simulink model "Linear_Model_Ters_Sarkac"  (R2022a)
settings: Solver=ode4  StartTime=0.0  StopTime=20  FixedStep=1/1000  RelTol=1e-3
InitFcn:
  | Sarkac_Parametrelerini_Yukle
values from neighbouring files (symbols this model uses):
  A = [0      1              0           0 ... (first row only)    [Sarkac_Parametrelerini_Yukle.m]
  B = [     0 ... (first row only)    [Sarkac_Parametrelerini_Yukle.m]
  Baslangic_Degerleri_Lin = [0,0,deg2rad(15),0]    [Sarkac_Parametrelerini_Yukle.m]
  C = eye(4)    [Sarkac_Parametrelerini_Yukle.m]
  D = zeros(4,1)    [Sarkac_Parametrelerini_Yukle.m]
  LQR_Katsayi_Matrisi = K    [Sarkac_Parametrelerini_Yukle.m]
libraries: simulink_extras x2, vrlib x1
settings Model: Creator=Fatabi  LastModifiedBy=Fatabi
settings SolverCC: AlgebraicLoopSolver=TrustRegion
settings DebuggingCC: UnconnectedInputMsg=warning  UnconnectedOutputMsg=warning  UnconnectedLineMsg=warning  SFMachineParentedDataDiag=warning

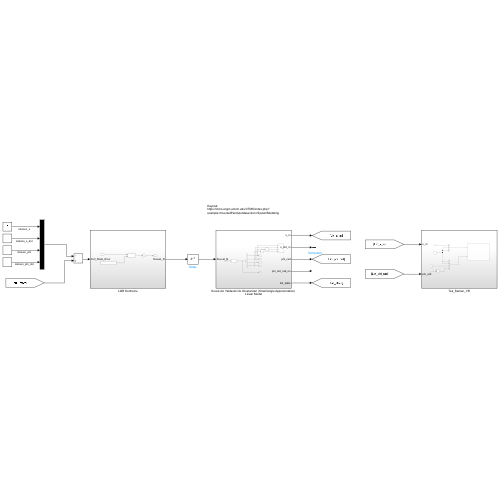
[thumbnail: Simulink's stored preview of the top-level diagram]
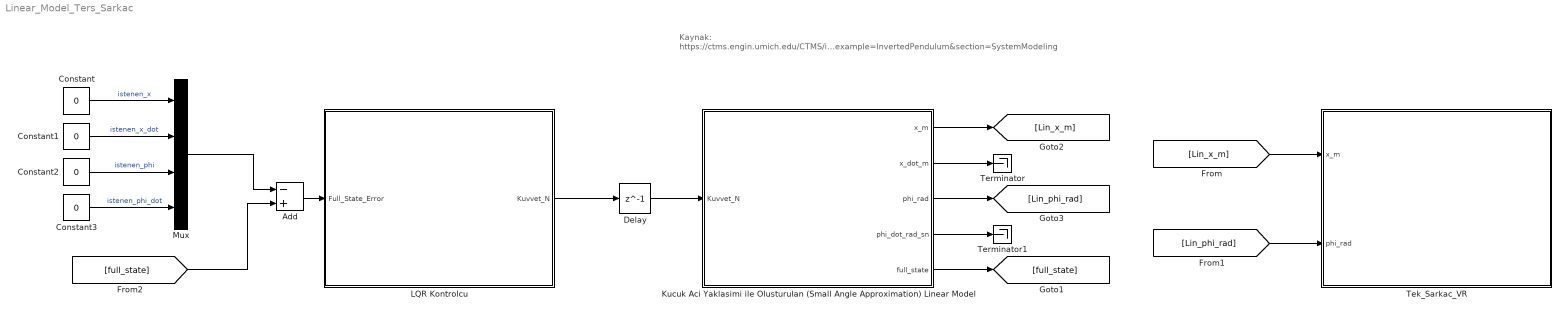
== system Linear_Model_Ters_Sarkac ==
  note: Kaynak:
      | https://ctms.engin.umich.edu/CTMS/index.php?example=InvertedPendulum&section=SystemModeling
  Add : Sum  Inputs=-+
  Constant{,1..3} (4 alike) : Constant  Value=0
  Delay : Delay  DelayLength=1
  Kucuk Aci Yaklasimi ile Olusturulan (Small Angle Approximation) Linear Model : Subsystem
  LQR Kontrolcu : Subsystem
  Mux : Mux
  "Tek_Sarkac_VR " : Subsystem
  Terminator : Terminator
  Terminator1 : Terminator
  wires:
  Kucuk Aci Yaklasimi ile Olusturulan (Small Angle Approximation) Linear Model/1(x_m) -> [Lin_x_m]
  Kucuk Aci Yaklasimi ile Olusturulan (Small Angle Approximation) Linear Model/3(phi_rad) -> [Lin_phi_rad]
  [Lin_x_m] -> "Tek_Sarkac_VR "/1(x_m)
  [Lin_phi_rad] -> "Tek_Sarkac_VR "/2("phi_rad ")
  Kucuk Aci Yaklasimi ile Olusturulan (Small Angle Approximation) Linear Model/2(x_dot_m) -> Terminator/1
  Kucuk Aci Yaklasimi ile Olusturulan (Small Angle Approximation) Linear Model/4(phi_dot_rad_sn) -> Terminator1/1
  Kucuk Aci Yaklasimi ile Olusturulan (Small Angle Approximation) Linear Model/5(full_state) -> [full_state]
  [full_state] -> Add/2
  Constant1/1 -> Mux/2  "istenen_x_dot"
  Constant/1 -> Mux/1  "istenen_x"
  Constant2/1 -> Mux/3  "istenen_phi"
  Constant3/1 -> Mux/4  "istenen_phi_dot"
  Mux/1 -> Add/1
  Add/1 -> LQR Kontrolcu/1(Full_State_Error)
  LQR Kontrolcu/1(Kuvvet_N) -> Delay/1
  Delay/1 -> Kucuk Aci Yaklasimi ile Olusturulan (Small Angle Approximation) Linear Model/1(Kuvvet_N)

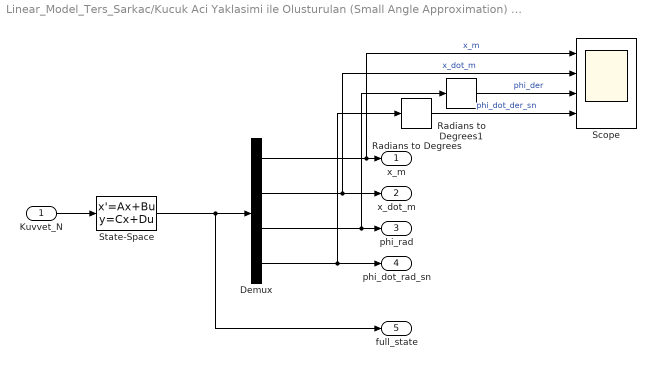
== system Linear_Model_Ters_Sarkac/Kucuk Aci Yaklasimi ile Olusturulan (Small Angle Approximation) Linear Model ==
  Kuvvet_N : Inport
  Demux : Demux
  Radians to Degrees : simulink_extras/Transformations/Radians to Degrees
  Radians to Degrees1 : simulink_extras/Transformations/Radians to Degrees
  Scope : Scope  NumInputPorts=4
  State-Space : StateSpace  A=A  B=B  C=C  D=D  InitialCondition=Baslangic_Degerleri_Lin
  x_m : Outport
  x_dot_m : Outport  Port=2
  phi_rad : Outport  Port=3
  phi_dot_rad_sn : Outport  Port=4
  full_state : Outport  Port=5
  wires:
  Demux/1 -> Scope/1, x_m/1  "x_m"
  Kuvvet_N/1 -> State-Space/1
  Demux/3 -> Radians to Degrees1/1, phi_rad/1
  Demux/4 -> phi_dot_rad_sn/1, Radians to Degrees/1
  Demux/2 -> x_dot_m/1, Scope/2  "x_dot_m"
  State-Space/1 -> full_state/1, Demux/1
  Radians to Degrees/1 -> Scope/4  "phi_dot_der_sn"
  Radians to Degrees1/1 -> Scope/3  "phi_der"

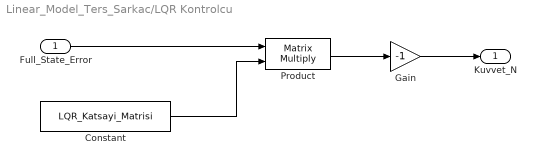
== system Linear_Model_Ters_Sarkac/LQR Kontrolcu ==
  Full_State_Error : Inport
  Constant : Constant  Value=LQR_Katsayi_Matrisi
  Gain : Gain  Gain=-1
  Product : Product  Multiplication=Matrix(*)
  Kuvvet_N : Outport
  wires:
  Constant/1 -> Product/2
  Full_State_Error/1 -> Product/1
  Product/1 -> Gain/1
  Gain/1 -> Kuvvet_N/1

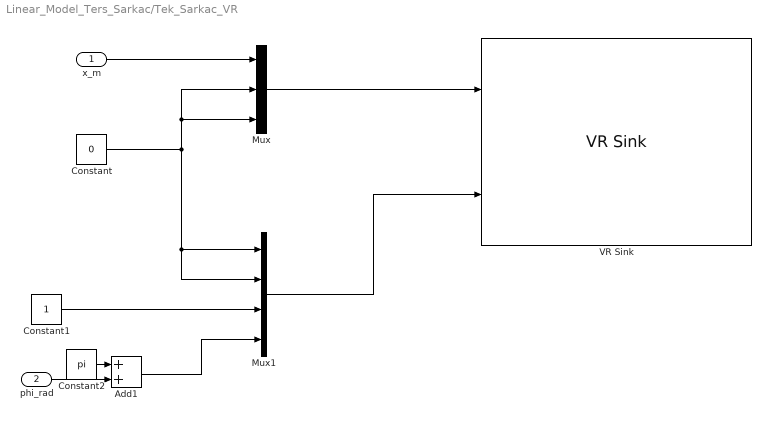
== system Linear_Model_Ters_Sarkac/Tek_Sarkac_VR  ==
  x_m : Inport
  "phi_rad " : Inport  Port=2
  Add1 : Sum
  Constant : Constant  Value=0
  Constant1 : Constant
  Constant2 : Constant  Value=pi
  Mux : Mux  Inputs=3
  Mux1 : Mux
  VR Sink : vrlib/VR Sink  InstantiateOnLoad=on  SampleTime=0.02  ViewEnable=on  RemoteChange=off  RemoteView=off  FieldsWritten=Kutu.translation.3.1.1.double#Mentese1.rotation.4.1.1.double  WorldFileName=sarkac.wrl  AutoView=off  VideoDimensions=[]  AllowVariableSize=off  FigureProperties="{'Position', 'Name', 'Viewpoint', 'CameraBound', 'CameraDirection', 'CameraPosition', 'CameraUpVector', 'ZoomFactor', 'Antialiasing', 'Headlight', 'Lighting', 'NavPanel', 'Sound', 'StatusBar', 'Stereo3D', 'Stereo3DCameraOffset', 'Stereo3DHIT', 'ToolBar', 'Textures', 'Transparency', 'Triad', 'Wireframe', 'NavZones', 'NavMode', 'NavSpeed', 'CaptureFileFormat', 'CaptureFileName', 'Record2DCompressMethod', 'Record2DCompressQuality', 'Record2D', 'Record2DFileName', 'Record2DFPS'; [9.9300000000000000e+02   8.4000000000000000e+01   9.2700000000000000e+02   9.4400000000000000e+02], '', '_untitled_1', 'on', [0.0000000000000000e+00   0.0000000000000000e+00  -1.0000000000000000e+00], [0.0000000000000000e+00   0.0000000000000000e+00  -3.0000000000000000e+00], [0.0000000000000000e+00   1.0000000000000000e+00   0.0000000000000000e+00], [1.0000000000000000e+00], 'on', 'on', 'on', 'halfbar', 'on', 'on', 'off', [1.0000000149011612e-01], [0.0000000000000000e+00], 'on', 'on', 'on', 'none', 'off', 'off', 'fly', 'normal', 'tif', '%f_anim_%n.tif', 'auto', [7.5000000000000000e+01], 'off', '%f_anim_%n.avi', 'auto'}"
  wires:
  x_m/1 -> Mux/1
  Constant/1 -> Mux/3, Mux/2, Mux1/2, Mux1/1
  "phi_rad "/1 -> Add1/2
  Constant1/1 -> Mux1/3
  Mux/1 -> VR Sink/1
  Mux1/1 -> VR Sink/2
  Constant2/1 -> Add1/1
  Add1/1 -> Mux1/4
